simulink model "amk_eff_estimator"  (R2024b)
settings: Solver=FixedStepAuto  StartTime=0.0  StopTime=10.0  RelTol=1e-3
model workspace (MAT data in the model file):
  AMKData.Shaft_Torque = [0 0 0 0 0 0 0 0 0 0 0 0 ... (4221 elements, 201x21)]
  AMKData.Vd_RMS = [-3.00349718007e-06 -0.000300349718007 -0.000600699436014 -0.000901049154021 -0.00120139887203 -0.00150174859004 -0.00180209830804 -0.00210244802605 -0.00240279774406 -0.00270314746206 -0.00300349718007 -0.00330384689808 ... (4221 elements, 201x21)]
  AMKData.Iq_RMS = [0 0 0 0 0 0 0 0 0 0 0 0 ... (4221 elements, 201x21)]
  AMKData.Electromagnetic_Torque = [0 0 0 0 0 0 0 0 0 0 0 0 ... (4221 elements, 201x21)]
  AMKData.Stator_Copper_Loss = [0 4.81312208602e-05 0.000192524883441 0.000433180987742 0.000770099533764 0.00120328052151 0.00173272395097 0.00235842982215 0.00308039813505 0.00389862888968 0.00481312208602 0.00582387772409 ... (4221 elements, 201x21)]
  AMKData.Total_Loss = [0 1.78584684769 3.64312606164 5.57183440859 7.57197019267 9.64353223877 11.7865196458 14.0009316828 16.2867677349 18.6440272718 21.0727098272 23.5728149849 ... (4221 elements, 201x21)]
  AMKData.Voltage_Phase_RMS = [0.0175468831209 1.75468831209 3.50937662418 5.26406493627 7.01875324836 8.77344156045 10.5281298725 12.2828181846 14.0375064967 15.7921948088 17.5468831209 19.301571433 ... (4221 elements, 201x21)]
  AMKData.Magnet_Loss = [0 0.000102129338713 0.000402651060243 0.000898331910851 0.00158747602166 0.00246890827873 0.00354172758693 0.00480520299395 0.00625871969102 0.00790174725718 0.00973381937651 0.0117545200864 ... (4221 elements, 201x21)]
  AMKData.Stator_Current_Phase_Peak = [0 0 0 0 0 0 0 0 0 0 0 0 ... (4221 elements, 201x21)]
  AMKData.Power_Factor = [0 0 0 0 0 0 0 0 0 0 0 0 ... (4221 elements, 201x21)]
  AMKData.Voltage_Line_RMS = [0.0175468831209 1.75468831209 3.50937662418 5.26406493627 7.01875324836 8.77344156045 10.5281298725 12.2828181846 14.0375064967 15.7921948088 17.5468831209 19.301571433 ... (4221 elements, 201x21)]
  AMKData.Vd_Peak = [-4.24758644661e-06 -0.000424758644661 -0.000849517289321 -0.00127427593398 -0.00169903457864 -0.0021237932233 -0.00254855186796 -0.00297331051262 -0.00339806915728 -0.00382282780195 -0.00424758644661 -0.00467234509127 ... (4221 elements, 201x21)]
  AMKData.Stator_Current_Line_RMS = [0 0 0 0 0 0 0 0 0 0 0 0 ... (4221 elements, 201x21)]
  AMKData.Stator_Current_Line_Peak = [0 0 0 0 0 0 0 0 0 0 0 0 ... (4221 elements, 201x21)]
  AMKData.Iron_Loss = [0 0.952363253799 1.97586421903 3.07050289569 4.23627928378 5.4731933833 6.78124519425 8.16043471664 9.61076195045 11.1322268957 12.7248295524 14.3885699205 ... (4221 elements, 201x21)]
  AMKData.Voltage_Phase_Peak = [0.024815040087 2.48150400869 4.96300801739 7.44451202608 9.92601603478 12.4075200435 14.8890240522 17.3705280609 19.8520320696 22.3335360782 24.8150400869 27.2965440956 ... (4221 elements, 201x21)]
  AMKData.Stator_Current_Phase_RMS = [0 0 0 0 0 0 0 0 0 0 0 0 ... (4221 elements, 201x21)]
  AMKData.Iq_Peak = [0 0 0 0 0 0 0 0 0 0 0 0 ... (4221 elements, 201x21)]
  AMKData.Voltage_Line_Peak = [0.024815040087 2.48150400869 4.96300801739 7.44451202608 9.92601603478 12.4075200435 14.8890240522 17.3705280609 19.8520320696 22.3335360782 24.8150400869 27.2965440956 ... (4221 elements, 201x21)]
  AMKData.Mechanical_Loss = [0 0.833333333333 1.66666666667 2.5 3.33333333333 4.16666666667 5 5.83333333333 6.66666666667 7.5 8.33333333333 9.16666666667 ... (4221 elements, 201x21)]
  AMKData.Id_RMS = [0 0 0 0 0 0 0 0 0 0 0 0 ... (4221 elements, 201x21)]
  AMKData.Id_Peak = [0 0 0 0 0 0 0 0 0 0 0 0 ... (4221 elements, 201x21)]
  AMKData.Vq_RMS = [0.0175468828638 1.75468828638 3.50937657277 5.26406485915 7.01875314554 8.77344143192 10.5281297183 12.2828180047 14.0375062911 15.7921945775 17.5468828638 19.3015711502 ... (4221 elements, 201x21)]
  AMKData.Frequency = [0.0833333333333 8.33333333333 16.6666666667 25 33.3333333333 41.6666666667 50 58.3333333333 66.6666666667 75 83.3333333333 91.6666666667 ... (4221 elements, 201x21)]
  AMKData.Vq_Peak = [0.0248150397234 2.48150397234 4.96300794468 7.44451191702 9.92601588936 12.4075198617 14.889023834 17.3705278064 19.8520317787 22.3335357511 24.8150397234 27.2965436958 ... (4221 elements, 201x21)]
  AMKData.Speed = [0 100 200 300 400 500 600 700 800 900 1000 1100 ... (4221 elements, 201x21)]
  AMKData.MechanicalPower = [0 -1.78585102378 -3.64313458085 -5.57184743796 -7.57198789923 -9.64355478954 -11.7865472078 -14.0009644231 -16.2868058205 -18.6440708697 -21.0727591043 -23.5728701084 ... (4221 elements, 201x21)]
  AMKData.electricalPower = [0 -4.17608676728e-06 -8.51921348e-06 -1.30293725764e-05 -1.77065600928e-05 -2.2550773279e-05 -2.75620100307e-05 -3.27402686349e-05 -3.80855476578e-05 -4.35978458526e-05 -4.92771621374e-05 -5.51234955317e-05 ... (4221 elements, 201x21)]
  AMKData.amk_eff = [0.6 0.6 0.6 0.6 0.6 0.6 0.6 0.6 0.6 0.6 0.6 0.6 ... (4221 elements, 201x21)]
  AMKData.T_flat = [0 0 0 0 0 0 0 0 0 0 0 0 ... (4221 elements, 4221x1)]
  AMKData.S_flat = [0 100 200 300 400 500 600 700 800 900 1000 1100 ... (4221 elements, 4221x1)]
  AMKData.Eff_flat = [0.6 0.6 0.6 0.6 0.6 0.6 0.6 0.6 0.6 0.6 0.6 0.6 ... (4221 elements, 4221x1)]
  AMKData.F_eff = scatteredInterpolant
  AMKData.F_eff.Points = [0 0 0 0 0 0 0 0 0 0 0 0 ... (8442 elements, 4221x2)]
  AMKData.F_eff.Values = [0.6 0.6 0.6 0.6 0.6 0.6 0.6 0.6 0.6 0.6 0.6 0.6 ... (4221 elements, 4221x1)]
  AMKData.F_eff.Method = 'linear'
  AMKData.F_eff.ExtrapolationMethod = 'boundary'
  AMKData.MBD_Speed = [0 500 1000 1500 2000 2500 3000 3500 4000 4500 5000 5500 6000 6500 7000 7500 8000 8500 9000 9500 10000 10500 11000 11500 12000 12500 13000 13500 14000 14500 15000 15500 16000 16500 17000 17500 18000 18500 19000 19500 20000]
  AMKData.MBD_Torque = [0 1 2 3 4 5 6 7 8 9 10 11 12 13 14 15 16 17 18 19 20 21]
  AMKData.MBD_eff_perc = [60 60 60 60 60 60 60 60 60 60 60 60 ... (902 elements, 41x22)]
  AMKData.torq_testpoints = [0 0.212121212121 0.424242424242 0.636363636364 0.848484848485 1.06060606061 1.27272727273 1.48484848485 1.69696969697 1.90909090909 2.12121212121 2.33333333333 2.54545454545 2.75757575758 2.9696969697 3.18181818182 3.39393939394 3.60606060606 3.81818181818 4.0303030303 4.24242424242 4.45454545455 4.66666666667 4.87878787879 5.09090909091 5.30303030303 5.51515151515 5.72727272727 5.93939393939 6.15151515152 6.36363636364 6.57575757576 6.78787878788 7 7.21212121212 7.42424242424 7.63636363636 7.84848484848 8.06060606061 8.27272727273 8.48484848485 8.69696969697 8.90909090909 9.12121212121 9.33333333333 9.54545454545 9.75757575758 9.9696969697 10.1818181818 10.3939393939 10.6060606061 10.8181818182 11.0303030303 11.2424242424 11.4545454545 11.6666666667 11.8787878788 12.0909090909 12.303030303 12.5151515152 12.7272727273 12.9393939394 13.1515151515 13.3636363636 13.5757575758 13.7878787879 14 14.2121212121 14.4242424242 14.6363636364 14.8484848485 15.0606060606 15.2727272727 15.4848484848 15.696969697 15.9090909091 16.1212121212 16.3333333333 16.5454545455 16.7575757576 16.9696969697 17.1818181818 17.3939393939 17.6060606061 17.8181818182 18.0303030303 18.2424242424 18.4545454545 18.6666666667 18.8787878788 19.0909090909 19.303030303 19.5151515152 19.7272727273 19.9393939394 20.1515151515 20.3636363636 20.5757575758 20.7878787879 21]
  AMKData.speed_testpoints = [0 202.02020202 404.04040404 606.060606061 808.080808081 1010.1010101 1212.12121212 1414.14141414 1616.16161616 1818.18181818 2020.2020202 2222.22222222 2424.24242424 2626.26262626 2828.28282828 3030.3030303 3232.32323232 3434.34343434 3636.36363636 3838.38383838 4040.4040404 4242.42424242 4444.44444444 4646.46464646 4848.48484848 5050.50505051 5252.52525253 5454.54545455 5656.56565657 5858.58585859 6060.60606061 6262.62626263 6464.64646465 6666.66666667 6868.68686869 7070.70707071 7272.72727273 7474.74747475 7676.76767677 7878.78787879 8080.80808081 8282.82828283 8484.84848485 8686.86868687 8888.88888889 9090.90909091 9292.92929293 9494.94949495 9696.96969697 9898.98989899 10101.010101 10303.030303 10505.0505051 10707.0707071 10909.0909091 11111.1111111 11313.1313131 11515.1515152 11717.1717172 11919.1919192 12121.2121212 12323.2323232 12525.2525253 12727.2727273 12929.2929293 13131.3131313 13333.3333333 13535.3535354 13737.3737374 13939.3939394 14141.4141414 14343.4343434 14545.4545455 14747.4747475 14949.4949495 15151.5151515 15353.5353535 15555.5555556 15757.5757576 15959.5959596 16161.6161616 16363.6363636 16565.6565657 16767.6767677 16969.6969697 17171.7171717 17373.7373737 17575.7575758 17777.7777778 17979.7979798 18181.8181818 18383.8383838 18585.8585859 18787.8787879 18989.8989899 19191.9191919 19393.9393939 19595.959596 19797.979798 20000]
  AMKData.torq_xq = [0 0 0 0 0 0 0 0 0 0 0 0 ... (10000 elements, 100x100)]
  AMKData.speed_yq = [0 202.02020202 404.04040404 606.060606061 808.080808081 1010.1010101 1212.12121212 1414.14141414 1616.16161616 1818.18181818 2020.2020202 2222.22222222 ... (10000 elements, 100x100)]
  AMKData.eff_zq = [0.6 0.6 0.6 0.6 0.6 0.6 0.6 0.6 0.6 0.6 0.6 0.6 ... (10000 elements, 100x100)]
  dt = Simulink.Parameter
  dt.Value = 0.004
  dt.Complexity = 'real'
  dt.Dimensions = [1 1]
  dt.DataType = 'double'
settings Model: Creator=lukec  LastModifiedBy=lukec
settings OptimizationCC: DefaultParameterBehavior=Inlined  EnhancedBackFolding=on  PassReuseOutputArgsAs=Individual arguments  ZeroExternalMemoryAtStartup=off  ZeroInternalMemoryAtStartup=off  OptimizeBlockOrder=speed  DifferentSizesBufferReuse=on  OptimizationCustomize=off  EfficientTunableParamExpr=on
settings DebuggingCC: ParameterTunabilityLossMsg=error
settings HardwareCC: ProdBitPerPointer=32  ProdBitPerSizeT=32  ProdBitPerPtrDiffT=32  ProdLargestAtomicInteger=Long  ProdLargestAtomicFloat=Double  ProdWordSize=32  ProdHWDeviceType=ARM Compatible->ARM Cortex-M
settings SFSimCC: MATLABDynamicMemAlloc=off
settings RTWCC: Description=Embedded Coder  SystemTargetFile=ert.tlc  GenCodeOnly=on  PackageGeneratedCodeAndArtifacts=on  TemplateMakefile=ert_default_tmf  Toolchain=CMake  TargetLang=C++  HalideCodeGeneration=on
settings CodeAppCC: ForceParamTrailComments=on  IgnoreCustomStorageClasses=off  MaxIdLength=255  OperatorAnnotations=on  SimulinkDataObjDesc=on  SFDataObjDesc=on  InsertBlockDesc=on
settings ERTTargetCC: TargetLangStandard=C++17 (ISO)  CodeInterfacePackaging=C++ class  RootIOFormat=Structure reference  ERTCustomFileTemplate=example_file_process.tlc  ArrayContainerType=std::array

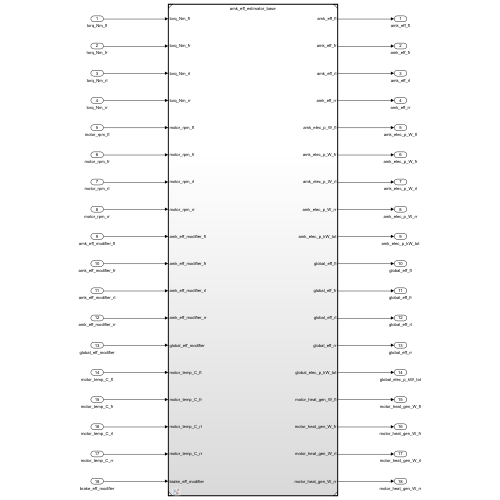
[thumbnail: Simulink's stored preview of the top-level diagram]
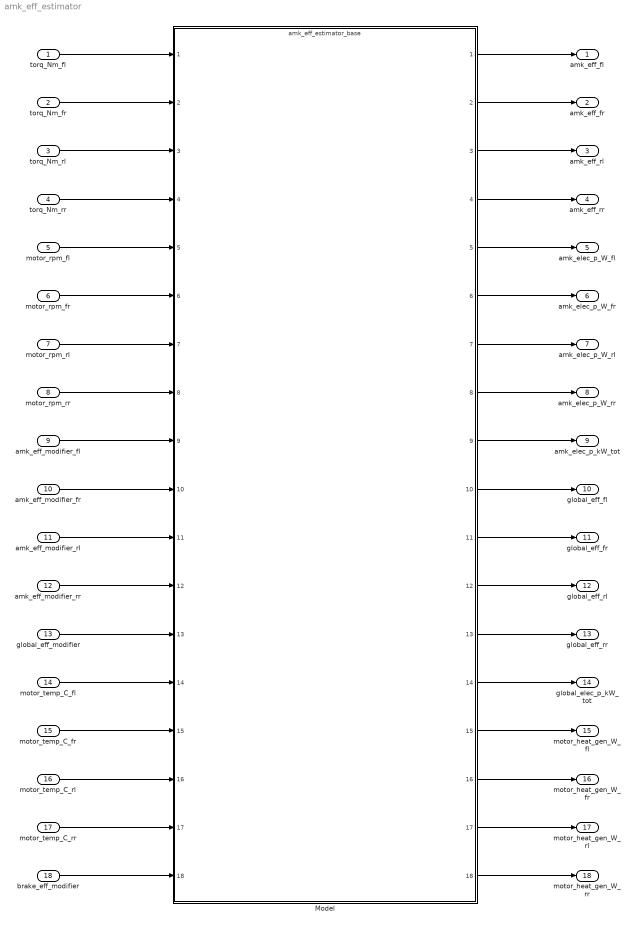
== system amk_eff_estimator ==
  torq_Nm_fl : Inport
  torq_Nm_fr : Inport  Port=2
  torq_Nm_rl : Inport  Port=3
  torq_Nm_rr : Inport  Port=4
  motor_rpm_fl : Inport  Port=5
  motor_rpm_fr : Inport  Port=6
  motor_rpm_rl : Inport  Port=7
  motor_rpm_rr : Inport  Port=8
  amk_eff_modifier_fl : Inport  Port=9
  amk_eff_modifier_fr : Inport  Port=10
  amk_eff_modifier_rl : Inport  Port=11
  amk_eff_modifier_rr : Inport  Port=12
  global_eff_modifier : Inport  Port=13
  motor_temp_C_fl : Inport  Port=14
  motor_temp_C_fr : Inport  Port=15
  motor_temp_C_rl : Inport  Port=16
  motor_temp_C_rr : Inport  Port=17
  brake_eff_modifier : Inport  Port=18
  Model : ModelReference  ModelNameDialog=amk_eff_estimator_base.slx  SimulationMode=Normal  ModelReferenceVersion=1.32
  amk_eff_fl : Outport
  amk_eff_fr : Outport  Port=2
  amk_eff_rl : Outport  Port=3
  amk_eff_rr : Outport  Port=4
  amk_elec_p_W_fl : Outport  Port=5
  amk_elec_p_W_fr : Outport  Port=6
  amk_elec_p_W_rl : Outport  Port=7
  amk_elec_p_W_rr : Outport  Port=8
  amk_elec_p_kW_tot : Outport  Port=9
  global_eff_fl : Outport  Port=10
  global_eff_fr : Outport  Port=11
  global_eff_rl : Outport  Port=12
  global_eff_rr : Outport  Port=13
  global_elec_p_kW_tot : Outport  Port=14
  motor_heat_gen_W_fl : Outport  Port=15
  motor_heat_gen_W_fr : Outport  Port=16
  motor_heat_gen_W_rl : Outport  Port=17
  motor_heat_gen_W_rr : Outport  Port=18
  wires:
  torq_Nm_fl/1 -> Model/1
  torq_Nm_fr/1 -> Model/2
  torq_Nm_rl/1 -> Model/3
  motor_rpm_fr/1 -> Model/6
  motor_rpm_fl/1 -> Model/5
  torq_Nm_rr/1 -> Model/4
  motor_rpm_rr/1 -> Model/8
  amk_eff_modifier_fl/1 -> Model/9
  motor_rpm_rl/1 -> Model/7
  Model/1 -> amk_eff_fl/1
  Model/2 -> amk_eff_fr/1
  Model/3 -> amk_eff_rl/1
  Model/4 -> amk_eff_rr/1
  Model/5 -> amk_elec_p_W_fl/1
  Model/6 -> amk_elec_p_W_fr/1
  Model/7 -> amk_elec_p_W_rl/1
  Model/8 -> amk_elec_p_W_rr/1
  Model/9 -> amk_elec_p_kW_tot/1
  amk_eff_modifier_fr/1 -> Model/10
  amk_eff_modifier_rl/1 -> Model/11
  amk_eff_modifier_rr/1 -> Model/12
  global_eff_modifier/1 -> Model/13
  Model/10 -> global_eff_fl/1
  Model/11 -> global_eff_fr/1
  Model/12 -> global_eff_rl/1
  Model/13 -> global_eff_rr/1
  Model/14 -> global_elec_p_kW_tot/1
  motor_temp_C_fl/1 -> Model/14
  motor_temp_C_fr/1 -> Model/15
  motor_temp_C_rl/1 -> Model/16
  motor_temp_C_rr/1 -> Model/17
  Model/15 -> motor_heat_gen_W_fl/1
  Model/16 -> motor_heat_gen_W_fr/1
  Model/17 -> motor_heat_gen_W_rl/1
  Model/18 -> motor_heat_gen_W_rr/1
  brake_eff_modifier/1 -> Model/18
